simulink model "untitled"  (R2025b)
settings: Solver=FixedStepAuto  StartTime=0.0  StopTime=100  FixedStep=.01  RelTol=1e-3
undefined symbols (not defined in the file or in its folder): battery_builder_rtmsupport, gcbh
libraries: Batteries_lib x15, nesl_utility x5, fl_lib x4, ee_lib x1
(part 2 of 2)

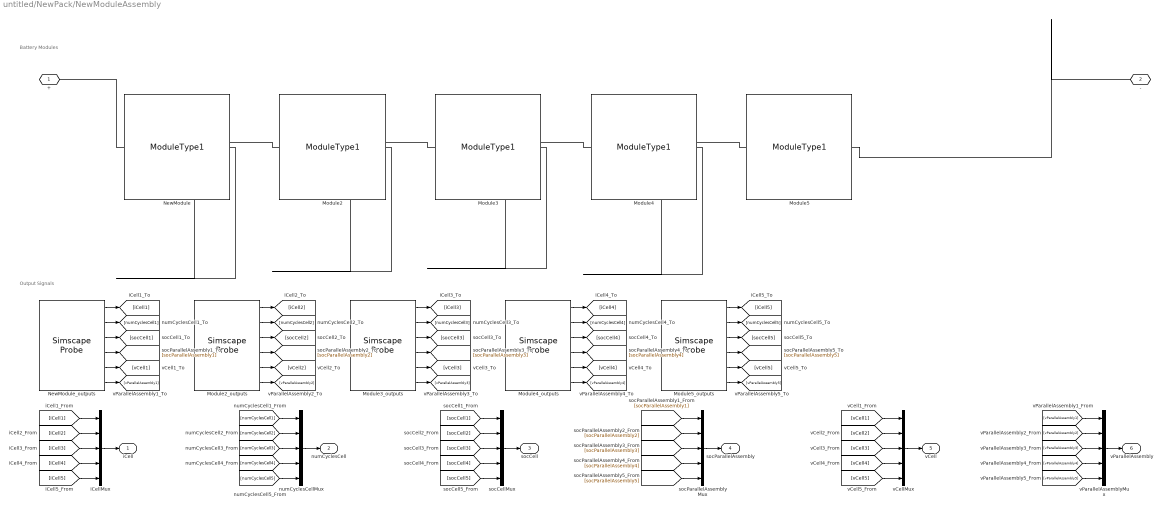
== system untitled/NewPack/NewModuleAssembly ==
  note: Battery Modules
  note: Output Signals
  Module{2..5} (4 alike) : Batteries_lib/Modules/ModuleType1  SOC_vecCell=[0, .01, .02, .03, .04, .05, .06, .07, .08, .09, .1, .11, .12, .13, .14, .15, .16, .17, .18, .19, .2, .21, .22, .23, .24, .25, .26, .27, .28, .29, .3, .31, .32, .33, .34, .35, .36, .37, .38, .39, .4, .41, .42, .43, .44, .45, .46, .47, .48, .49, .5, .51, .52, .53, .54, .55, .56, .57, .58, .59, .6, .61, .62, .63, .64, .65, .66, .67, .68, .69, .7, .71, .72, .73, .74, .75, .76, .77, .78, .79, .8, .81, .82, .83, .84, .85, .86, .87, .88, .89, .9, .91, .92, .93, .94, .95, .96, .97, .98, .99, 1]  V0_vecCell=[3.17242, 3.18272, 3.19302, 3.20331, 3.21361, 3.22391, 3.23421, 3.24451, 3.25481, 3.2651, 3.2754, 3.2857, 3.296, 3.3063, 3.31659, 3.32689, 3.33719, 3.34749, 3.35779, 3.36809, 3.37838, 3.38868, 3.39898, 3.40928, 3.41958, 3.42988, 3.44017, 3.45047, 3.46077, 3.47107, 3.48137, 3.49166, 3.50196, 3.51226, 3.52256, 3.53286, 3.54316, 3.55345, 3.56375, 3.57405, 3.58435, 3.59465, 3.60495, 3.61524, 3.62554, 3.63584, 3.64614, 3.65644, 3.66673, 3.67703, 3.68733, 3.69763, 3.71041, 3.72113, 3.72997, 3.73882, 3.74912, 3.75936, 3.76951, 3.7791, 3.78865, 3.79787, 3.80709, 3.8161, 3.82509, 3.83409, 3.84308, 3.85207, 3.86107, 3.87006, 3.87901, 3.88831, 3.89824, 3.90887, 3.91951, 3.93012, 3.94073, 3.95138, 3.96184, 3.97226, 3.98268, 3.99311, 4.0032, 4.01221, 4.01944, 4.02668, 4.03286, 4.03874, 4.04383, 4.0488, 4.05377, 4.05873, 4.06312, 4.06753, 4.07333, 4.08117, 4.08904, 4.09911, 4.11111, 4.13802, 4.16831] V  V_rangeCell=[2.25, Inf] V  R0_vecCell=[.02095, .01921, .01774, .0166, .01557, .01469, .01398, .01338, .01283, .01239, .01196, .01155, .01116, .01079, .01042, .01007, .00974, .00949, .00924, .009, .00876, .00855, .00843, .00832, .00826, .00825, .00825, .00826, .00827, .00828, .0083, .00834, .00838, .00842, .00848, .00855, .00863, .00871, .00879, .00887, .00895, .00903, .00911, .00918, .00925, .00931, .00938, .00946, .00953, .00961, .00968, .00976, .00991, .01, .01003, .01006, .01013, .01022, .0103, .01037, .01043, .01049, .01055, .01061, .01066, .01072, .01077, .01082, .01088, .01093, .01099, .01105, .01114, .01125, .01136, .01148, .01161, .01175, .01188, .01202, .01215, .01228, .01241, .01253, .01261, .01269, .01275, .0128, .01285, .01289, .01294, .01298, .01296, .01292, .01292, .01288, .01282, .0128, .01232, .01214, .00952] Ohm  AHCell=4.493 A*hr  extrapolation_optionCell=simscape.enum.extrapolation.nearest  P=1  S=13  iCell_specify=off  iCell_priority=None  iCell=0 A  iCell_nominal_specify=off  iCell_nominal_value=1  iCell_nominal_unit=A  vCell_specify=off  vCell_priority=None  vCell=0 V  vCell_nominal_specify=off  vCell_nominal_value=1  vCell_nominal_unit=V  socCell_specify=off  socCell_priority=High  socCell=1  socCell_nominal_specify=off  socCell_nominal_value=1  socCell_nominal_unit=1  numCyclesCell_specify=off  numCyclesCell_priority=High  numCyclesCell=0  numCyclesCell_nominal_specify=off  numCyclesCell_nominal_value=1  numCyclesCell_nominal_unit=1  vParallelAssembly_specify=off  vParallelAssembly_priority=None  vParallelAssembly=repmat(0, 13, 1) V  vParallelAssembly_nominal_specify=off  vParallelAssembly_nominal_value=1  vParallelAssembly_nominal_unit=V  socParallelAssembly_specify=off  socParallelAssembly_priority=None  socParallelAssembly=repmat(1, 13, 1)  socParallelAssembly_nominal_specify=off  socParallelAssembly_nominal_value=1  socParallelAssembly_nominal_unit=1
      settings: InternalSimscapePortConfiguration="{\"Bottom\":[{\"id\":\"n\",\"label\":\"-\",\"type\":\"foundation.electrical.electrical\"}],\"Left\":[],\"Right\":[],\"Top\":[{\"id\":\"p\",\"label\":\"+\",\"type\":\"foundation.electrical.electrical\"}]}"
  Module2_outputs : SimscapeProbe  BoundBlock=227  Variables="{\"iCell\":{\"Probing\":\"ON\"},\"numCyclesCell\":{\"Probing\":\"ON\"},\"socCell\":{\"Probing\":\"ON\"},\"socParallelAssembly\":{\"Probing\":\"ON\"},\"vCell\":{\"Probing\":\"ON\"},\"vParallelAssembly\":{\"Probing\":\"ON\"}}"
  Module3_outputs : SimscapeProbe  BoundBlock=229  Variables="{\"iCell\":{\"Probing\":\"ON\"},\"numCyclesCell\":{\"Probing\":\"ON\"},\"socCell\":{\"Probing\":\"ON\"},\"socParallelAssembly\":{\"Probing\":\"ON\"},\"vCell\":{\"Probing\":\"ON\"},\"vParallelAssembly\":{\"Probing\":\"ON\"}}"
  Module4_outputs : SimscapeProbe  BoundBlock=231  Variables="{\"iCell\":{\"Probing\":\"ON\"},\"numCyclesCell\":{\"Probing\":\"ON\"},\"socCell\":{\"Probing\":\"ON\"},\"socParallelAssembly\":{\"Probing\":\"ON\"},\"vCell\":{\"Probing\":\"ON\"},\"vParallelAssembly\":{\"Probing\":\"ON\"}}"
  Module5_outputs : SimscapeProbe  BoundBlock=233  Variables="{\"iCell\":{\"Probing\":\"ON\"},\"numCyclesCell\":{\"Probing\":\"ON\"},\"socCell\":{\"Probing\":\"ON\"},\"socParallelAssembly\":{\"Probing\":\"ON\"},\"vCell\":{\"Probing\":\"ON\"},\"vParallelAssembly\":{\"Probing\":\"ON\"}}"
  NewModule : Batteries_lib/Modules/ModuleType1  SOC_vecCell=[0, .01, .02, .03, .04, .05, .06, .07, .08, .09, .1, .11, .12, .13, .14, .15, .16, .17, .18, .19, .2, .21, .22, .23, .24, .25, .26, .27, .28, .29, .3, .31, .32, .33, .34, .35, .36, .37, .38, .39, .4, .41, .42, .43, .44, .45, .46, .47, .48, .49, .5, .51, .52, .53, .54, .55, .56, .57, .58, .59, .6, .61, .62, .63, .64, .65, .66, .67, .68, .69, .7, .71, .72, .73, .74, .75, .76, .77, .78, .79, .8, .81, .82, .83, .84, .85, .86, .87, .88, .89, .9, .91, .92, .93, .94, .95, .96, .97, .98, .99, 1]  V0_vecCell=[3.17242, 3.18272, 3.19302, 3.20331, 3.21361, 3.22391, 3.23421, 3.24451, 3.25481, 3.2651, 3.2754, 3.2857, 3.296, 3.3063, 3.31659, 3.32689, 3.33719, 3.34749, 3.35779, 3.36809, 3.37838, 3.38868, 3.39898, 3.40928, 3.41958, 3.42988, 3.44017, 3.45047, 3.46077, 3.47107, 3.48137, 3.49166, 3.50196, 3.51226, 3.52256, 3.53286, 3.54316, 3.55345, 3.56375, 3.57405, 3.58435, 3.59465, 3.60495, 3.61524, 3.62554, 3.63584, 3.64614, 3.65644, 3.66673, 3.67703, 3.68733, 3.69763, 3.71041, 3.72113, 3.72997, 3.73882, 3.74912, 3.75936, 3.76951, 3.7791, 3.78865, 3.79787, 3.80709, 3.8161, 3.82509, 3.83409, 3.84308, 3.85207, 3.86107, 3.87006, 3.87901, 3.88831, 3.89824, 3.90887, 3.91951, 3.93012, 3.94073, 3.95138, 3.96184, 3.97226, 3.98268, 3.99311, 4.0032, 4.01221, 4.01944, 4.02668, 4.03286, 4.03874, 4.04383, 4.0488, 4.05377, 4.05873, 4.06312, 4.06753, 4.07333, 4.08117, 4.08904, 4.09911, 4.11111, 4.13802, 4.16831] V  V_rangeCell=[2.25, Inf] V  R0_vecCell=[.02095, .01921, .01774, .0166, .01557, .01469, .01398, .01338, .01283, .01239, .01196, .01155, .01116, .01079, .01042, .01007, .00974, .00949, .00924, .009, .00876, .00855, .00843, .00832, .00826, .00825, .00825, .00826, .00827, .00828, .0083, .00834, .00838, .00842, .00848, .00855, .00863, .00871, .00879, .00887, .00895, .00903, .00911, .00918, .00925, .00931, .00938, .00946, .00953, .00961, .00968, .00976, .00991, .01, .01003, .01006, .01013, .01022, .0103, .01037, .01043, .01049, .01055, .01061, .01066, .01072, .01077, .01082, .01088, .01093, .01099, .01105, .01114, .01125, .01136, .01148, .01161, .01175, .01188, .01202, .01215, .01228, .01241, .01253, .01261, .01269, .01275, .0128, .01285, .01289, .01294, .01298, .01296, .01292, .01292, .01288, .01282, .0128, .01232, .01214, .00952] Ohm  AHCell=4.493 A*hr  extrapolation_optionCell=simscape.enum.extrapolation.nearest  P=1  S=13  iCell_specify=off  iCell_priority=None  iCell=0 A  iCell_nominal_specify=off  iCell_nominal_value=1  iCell_nominal_unit=A  vCell_specify=off  vCell_priority=None  vCell=0 V  vCell_nominal_specify=off  vCell_nominal_value=1  vCell_nominal_unit=V  socCell_specify=off  socCell_priority=High  socCell=1  socCell_nominal_specify=off  socCell_nominal_value=1  socCell_nominal_unit=1  numCyclesCell_specify=off  numCyclesCell_priority=High  numCyclesCell=0  numCyclesCell_nominal_specify=off  numCyclesCell_nominal_value=1  numCyclesCell_nominal_unit=1  vParallelAssembly_specify=off  vParallelAssembly_priority=None  vParallelAssembly=repmat(0, 13, 1) V  vParallelAssembly_nominal_specify=off  vParallelAssembly_nominal_value=1  vParallelAssembly_nominal_unit=V  socParallelAssembly_specify=off  socParallelAssembly_priority=None  socParallelAssembly=repmat(1, 13, 1)  socParallelAssembly_nominal_specify=off  socParallelAssembly_nominal_value=1  socParallelAssembly_nominal_unit=1
      settings: InternalSimscapePortConfiguration="{\"Bottom\":[{\"id\":\"n\",\"label\":\"-\",\"type\":\"foundation.electrical.electrical\"}],\"Left\":[],\"Right\":[],\"Top\":[{\"id\":\"p\",\"label\":\"+\",\"type\":\"foundation.electrical.electrical\"}]}"
  NewModule_outputs : SimscapeProbe  BoundBlock=235  Variables="{\"iCell\":{\"Probing\":\"ON\"},\"numCyclesCell\":{\"Probing\":\"ON\"},\"socCell\":{\"Probing\":\"ON\"},\"socParallelAssembly\":{\"Probing\":\"ON\"},\"vCell\":{\"Probing\":\"ON\"},\"vParallelAssembly\":{\"Probing\":\"ON\"}}"
  iCellMux : Mux  Inputs=5
  numCyclesCellMux : Mux  Inputs=5
  socCellMux : Mux  Inputs=5
  socParallelAssemblyMux : Mux  Inputs=5
  vCellMux : Mux  Inputs=5
  vParallelAssemblyMux : Mux  Inputs=5
  + : PMIOPort  Side=Left
  - : PMIOPort  Port=2  Side=Right
  iCell : Outport
  numCyclesCell : Outport  Port=2
  socCell : Outport  Port=3
  socParallelAssembly : Outport  Port=4
  vCell : Outport  Port=5
  vParallelAssembly : Outport  Port=6
  wires:
  NewModule_outputs/1 -> [iCell1]
  iCellMux/1 -> iCell/1
  [iCell1] -> iCellMux/1
  NewModule_outputs/2 -> [numCyclesCell1]
  numCyclesCellMux/1 -> numCyclesCell/1
  [numCyclesCell1] -> numCyclesCellMux/1
  NewModule_outputs/3 -> [socCell1]
  socCellMux/1 -> socCell/1
  [socCell1] -> socCellMux/1
  NewModule_outputs/4 -> [socParallelAssembly1]
  socParallelAssemblyMux/1 -> socParallelAssembly/1
  [socParallelAssembly1] -> socParallelAssemblyMux/1
  NewModule_outputs/5 -> [vCell1]
  vCellMux/1 -> vCell/1
  [vCell1] -> vCellMux/1
  NewModule_outputs/6 -> [vParallelAssembly1]
  vParallelAssemblyMux/1 -> vParallelAssembly/1
  [vParallelAssembly1] -> vParallelAssemblyMux/1
  Module2_outputs/1 -> [iCell2]
  [iCell2] -> iCellMux/2
  Module2_outputs/2 -> [numCyclesCell2]
  [numCyclesCell2] -> numCyclesCellMux/2
  Module2_outputs/3 -> [socCell2]
  [socCell2] -> socCellMux/2
  Module2_outputs/4 -> [socParallelAssembly2]
  [socParallelAssembly2] -> socParallelAssemblyMux/2
  Module2_outputs/5 -> [vCell2]
  [vCell2] -> vCellMux/2
  Module2_outputs/6 -> [vParallelAssembly2]
  [vParallelAssembly2] -> vParallelAssemblyMux/2
  Module3_outputs/1 -> [iCell3]
  [iCell3] -> iCellMux/3
  Module3_outputs/2 -> [numCyclesCell3]
  [numCyclesCell3] -> numCyclesCellMux/3
  Module3_outputs/3 -> [socCell3]
  [socCell3] -> socCellMux/3
  Module3_outputs/4 -> [socParallelAssembly3]
  [socParallelAssembly3] -> socParallelAssemblyMux/3
  Module3_outputs/5 -> [vCell3]
  [vCell3] -> vCellMux/3
  Module3_outputs/6 -> [vParallelAssembly3]
  [vParallelAssembly3] -> vParallelAssemblyMux/3
  Module4_outputs/1 -> [iCell4]
  [iCell4] -> iCellMux/4
  Module4_outputs/2 -> [numCyclesCell4]
  [numCyclesCell4] -> numCyclesCellMux/4
  Module4_outputs/3 -> [socCell4]
  [socCell4] -> socCellMux/4
  Module4_outputs/4 -> [socParallelAssembly4]
  [socParallelAssembly4] -> socParallelAssemblyMux/4
  Module4_outputs/5 -> [vCell4]
  [vCell4] -> vCellMux/4
  Module4_outputs/6 -> [vParallelAssembly4]
  [vParallelAssembly4] -> vParallelAssemblyMux/4
  Module5_outputs/1 -> [iCell5]
  [iCell5] -> iCellMux/5
  Module5_outputs/2 -> [numCyclesCell5]
  [numCyclesCell5] -> numCyclesCellMux/5
  Module5_outputs/3 -> [socCell5]
  [socCell5] -> socCellMux/5
  Module5_outputs/4 -> [socParallelAssembly5]
  [socParallelAssembly5] -> socParallelAssemblyMux/5
  Module5_outputs/5 -> [vCell5]
  [vCell5] -> vCellMux/5
  Module5_outputs/6 -> [vParallelAssembly5]
  [vParallelAssembly5] -> vParallelAssemblyMux/5
  connections:
  Module2/LConn1 -- NewModule/RConn1
  Module3/LConn1 -- Module2/RConn1
  Module4/LConn1 -- Module3/RConn1
  Module5/LConn1 -- Module4/RConn1
  NewModule/LConn1 -- +/RConn1
  Module5/RConn1 -- -/RConn1

== matlab function untitled/Charger/Charger_core ==
  settings: updateMethod=DISCRETE  sampleTime=0.01
  data: pack_meas input; I_chg_cmd output; enable input; I_limit input; P_chg_cmd output; mode output; V_set output; I_set output; done output
function [I_chg_cmd, P_chg_cmd, mode, V_set, I_set, done] = ...
        fcn(pack_meas, enable, I_limit)
%#codegen
%CHARGER_CORE  Generated by bcp.ChargerBuilder. Do not edit here.
%
%  Edit bcp.ChargerConfig (or the Charger tab of bcpApp) and re-insert the
%  block. Changes made in this window are overwritten by the next insert.
%
%  pack_meas indices are fixed by bcp.Signals:
%    1 V_pack  2 V_cell_min  3 V_cell_max  4 SOC_pack  5 SOC_min
%    6 SOC_max 7 I_pack (charge-positive)

P = struct( ...
        'Ts', 0.01, ...
        'SeriesCount', 14, ...
        'I_cc_A', 21.75, ...
        'I_taper_A', 1.125, ...
        'I_precharge_A', 2.25, ...
        'V_cv_cell', 4.2, ...
        'V_cv_pack', 58.8, ...
        'V_precharge_cell', 3, ...
        'V_recharge_cell', 4.05, ...
        'Kp_cell', 125, ...
        'Ki_cell', 250, ...
        'Kp_pack', 8.92857142857, ...
        'Ki_pack', 17.8571428571, ...
        't_term_s', 2, ...
        'ForceMode', 0);

%  The CV loop is handed the HIGHEST cell, not the pack average. On a pack
%  with real cell spread those are different constraints, and the per-cell
%  one is what keeps a cell out of over-voltage. See bcp_charger.
[I_chg_cmd, P_chg_cmd, mode, V_set, I_set, done] = bcp_charger( ...
    pack_meas(1), pack_meas(3), pack_meas(7), enable, I_limit, P);

%  Supply power ceiling, applied last so it cannot be reasoned around by the
%  control law: a real supply simply cannot deliver more than this.
if P_chg_cmd > 1278.9
    P_chg_cmd = 1278.9;
    if pack_meas(1) > 1
        I_chg_cmd = P_chg_cmd / pack_meas(1);
    end
end
end

== matlab function untitled/BMS/BMS_core ==
  settings: updateMethod=DISCRETE  sampleTime=0.01
  data: t input; P_load_cmd output; Vcell input; SOCcell input; Icell input; Tmax input; P_chg input; chg_done input; reset input; P_net_cmd output; chg_enable output; I_chg_limit output; pack_meas output; contactor output; state output; faults output; diag output
function [P_load_cmd, P_net_cmd, chg_enable, I_chg_limit, pack_meas, ...
          contactor, state, faults, diag] = ...
        fcn(t, Vcell, SOCcell, Icell, Tmax, P_chg, chg_done, reset)
%#codegen
%BMS_CORE  Generated by bcp.BmsBuilder. Do not edit here.
%
%  Edit bcp.BmsConfig / bcp.LoadSignal (or the Load and BMS tabs of bcpApp)
%  and re-insert the block. Changes made in this window are overwritten by
%  the next insert, and are invisible to the tests.
%
%  Sign convention inside this function: POSITIVE CURRENT = CHARGING.
%  Load power is DRAW-POSITIVE. The two meet at P_net_cmd.

MON = struct( ...
        'SeriesCount', 14, ...
        'I_sign', -1, ...
        'SOC_in_percent', false);
PRO = struct( ...
        'Ts', 0.01, ...
        'V_ov_trip', 4.25, ...
        'V_ov_clear', 4.1, ...
        'V_uv_trip', 2.45, ...
        'V_uv_clear', 2.8, ...
        't_v_trip', 0.5, ...
        'I_chg_trip', 25, ...
        'I_dch_trip', 248, ...
        't_i_trip', 0.1, ...
        'T_ot_trip', 60, ...
        'T_ot_clear', 50, ...
        'T_ut_trip', 0, ...
        't_T_trip', 5, ...
        'AutoRecover', true, ...
        't_recover', 2);
ARB = struct( ...
        'Ts', 0.01, ...
        'ChargeEnabled', true, ...
        'AllowConcurrent', false, ...
        't_quiet_s', 1, ...
        'SOC_stop', 0.95, ...
        'SOC_restart', 0.85, ...
        'V_recharge', 4.05, ...
        'I_chg_trip', 25, ...
        'I_chg_margin', 0.9, ...
        'I_chg_headroom_A', 5);
LOAD = struct( ...
        'Ts', 0.01, ...
        'Waveform', 3, ...
        'StartTime_s', 0, ...
        'StopTime_s', Inf, ...
        'Offset_W', 0, ...
        'Amplitude_W', 31250, ...
        'Frequency_Hz', 0.5, ...
        'Phase_deg', 0, ...
        'Duty_pct', 20, ...
        'Pmin_W', 0, ...
        'Pmax_W', 50000, ...
        'Slew_W_per_s', 0, ...
        'IdleThreshold_W', 5);
OUT_SIGN = 1;

%  1. Reduce the per-cell arrays to pack scalars.
pack_meas = bcp_pack_monitor(Vcell, SOCcell, Icell, MON);

%  2. What does the load waveform ask for at this instant?
[P_demand, demandPresent] = bcp_load_scheduler(t, LOAD);

%  3. Protection, on the pack extremes.
[contactor, chg_ok, dch_ok, state, faults, flags] = bcp_protection( ...
    pack_meas(2), pack_meas(3), Tmax, pack_meas(7), reset > 0.5, PRO);

%  4. A discharge inhibit has to inhibit the discharge. The load is the only
%     discharge path in this model, so dch_ok gates the load command -- and
%     the GATED value is what counts as "the load is active".
%
%     Order matters here. Feeding the ungated demand to the arbiter would
%     mean an under-voltage fault holds the load flag high, the arbiter sees
%     a busy load and refuses to charge, and the pack sits at its floor
%     forever -- deadlocked by its own protection, with a charger idle beside
%     it. The cure for under-voltage is a charge.
if dch_ok < 0.5
    P_load = 0;
else
    P_load = P_demand;
end
loadActive = double(abs(P_load) > LOAD.IdleThreshold_W);

%  5. Arbitrate. The load has already happened; this decides what is left.
[chg_enable, I_chg_limit, reason] = bcp_arbiter( ...
    loadActive, pack_meas(4), pack_meas(3), chg_ok, chg_done, ARB);

%  6. Shape the outputs.
P_load_cmd = OUT_SIGN * P_load;
P_net_cmd  = OUT_SIGN * (P_load - P_chg);

diag = [demandPresent; loadActive; reason; dch_ok; flags];
end
